simulink library "cdsDacKillTimed"  (Simulink 8.6)
settings: Solver=ode45  StartTime=0.0  StopTime=10.0  RelTol=1e-3
settings Model: Creator=rolf  LastModifiedBy=rolf

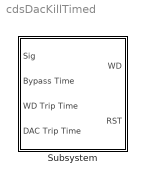
== system cdsDacKillTimed ==
  Subsystem : Subsystem

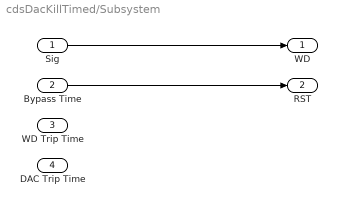
== system cdsDacKillTimed/Subsystem ==
  Sig : Inport
  Bypass Time : Inport  Port=2
  WD Trip Time : Inport  Port=3
  DAC Trip Time : Inport  Port=4
  WD : Outport
  RST : Outport  Port=2
  wires:
  Sig/1 -> WD/1
  Bypass Time/1 -> RST/1
